simulink model "general_SD_model"  (R2021a)
settings: Solver=ode45  StartTime=0.0  StopTime=tfinal  FixedStep=T  MaxStep=0.01  RelTol=1e-12  AbsTol=1e-12  EnableMultiTasking=on
values from neighbouring files (symbols this model uses):
  position_amplitude = 0.03    [lab3_part_c.m]    (also in paramGen.m = 0.1; paramGenPartE.m = 0.15; part_c.m)
  position_offset = 0.15    [lab3_part_c.m]    (also in paramGen.m; paramGenPartE.m = 0.1; part_c.m)
  T = 0.001    [lab3_part_c.m]    (also in paramGen.m; paramGenPartE.m; part_c.m)
libraries: cstblocks x5
settings Model: OrderedModelArguments=off  Creator=cnielsen  LastModifiedBy=Daniel Robson
settings SolverCC: AutoScaleAbsTol=off  AlgebraicLoopSolver=TrustRegion
settings DataIOCC: SaveFormat=Array  SignalLoggingSaveFormat=ModelDataLogs  SaveOutput=off  SaveTime=off  ReturnWorkspaceOutputs=off  Refine=5
settings OptimizationCC: ExpressionDepthLimit=2147483647  LifeSpan=inf
settings DebuggingCC: UnderspecifiedInitializationDetection=Classic  MergeDetectMultiDrivingBlocksExec=none  SolverPrmCheckMsg=warning  FcnCallInpInsideContextMsg=warning  StateNameClashWarn=warning  SFUnexpectedBacktrackingDiag=warning  SFNoUnconditionalDefaultTransitionDiag=warning  SFExecutionAtInitializationDiag=none  SFMachineParentedDataDiag=warning  ArithmeticOperatorsInVariantConditions=warning
settings HardwareCC: ProdBitPerPointer=32  ProdBitPerSizeT=32  ProdBitPerPtrDiffT=32  ProdLargestAtomicFloat=None  ProdIntDivRoundTo=Undefined  ProdEndianess=Unspecified  ProdWordSize=32  ProdHWDeviceType=32-bit Generic
settings ModelReferenceCC: PropagateSignalLabelsOutOfModel=off
settings SFSimCC: SimUseLocalCustomCode=off  CustomCodeUndefinedFunction=UseInterfaceOnly
settings RTWCC: RTWUseLocalCustomCode=off
settings CodeAppCC: StateflowObjectComments=on
settings GRTTargetCC: TargetLangStandard=C89/C90 (ANSI)  CombineOutputUpdateFcns=off  GRTInterface=on
settings ConfigComp: CovMetricSettings=dw  CovSaveCumulativeToWorkspaceVar=on  CovSaveSingleToWorkspaceVar=on  CovExternalEMLEnable=off

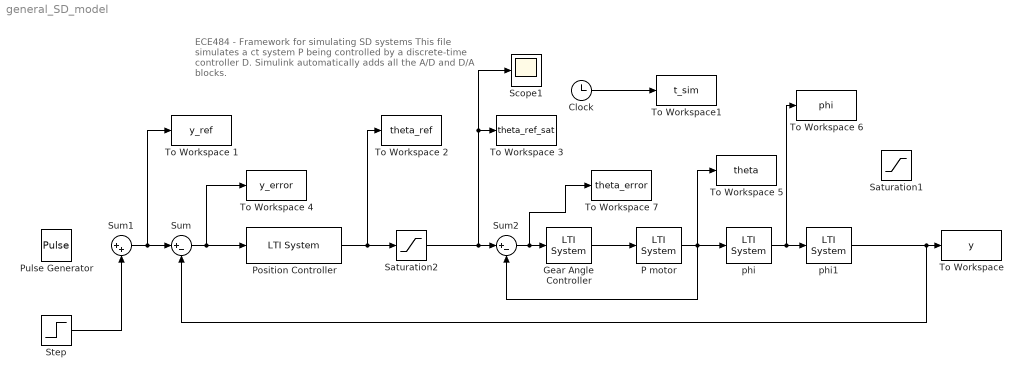
== system general_SD_model ==
  note: ECE484 - Framework for simulating SD systems
      | This file simulates a ct system P being controlled by a
      | discrete-time controller D. Simulink automatically adds all the
      | A/D and D/A blocks.
  Clock : Clock
  Gear Angle Controller : cstblocks/LTI System  sys=C_1  IC=[]
  P motor : cstblocks/LTI System  sys=P_motor  IC=[]
  Position Controller : cstblocks/LTI System  sys=C_2  IC=[]
  Pulse Generator : DiscretePulseGenerator  PulseType=Time based  Amplitude=position_amplitude  Period=20  PulseWidth=50  SampleTime=T
  Saturation1 : Saturate  UpperLimit=0.3916  LowerLimit=0
  Saturation2 : Saturate  UpperLimit=0.7  LowerLimit=-0.7
  Scope1 : Scope
  Step : Step  Time=0  After=position_offset  SampleTime=T
  Sum : Sum  Inputs=|+-
  Sum1 : Sum  Inputs=|++
  Sum2 : Sum  Inputs=|+-
  To Workspace : ToWorkspace  VariableName=y  SampleTime=T
  To Workspace 1 : ToWorkspace  VariableName=y_ref  SampleTime=T
  To Workspace 2 : ToWorkspace  VariableName=theta_ref  SampleTime=T
  To Workspace 3 : ToWorkspace  VariableName=theta_ref_sat  SampleTime=T
  To Workspace 4 : ToWorkspace  VariableName=y_error  SampleTime=T
  To Workspace 5 : ToWorkspace  VariableName=theta  SampleTime=T
  To Workspace 6 : ToWorkspace  VariableName=phi  SampleTime=T
  To Workspace 7 : ToWorkspace  VariableName=theta_error  SampleTime=T
  To Workspace1 : ToWorkspace  VariableName=t_sim  SampleTime=T
  phi : cstblocks/LTI System  sys=THETA_TO_PHI  IC=[]
  phi1 : cstblocks/LTI System  sys=PHI_TO_Y  IC=[]
  wires:
  Clock/1 -> To Workspace1/1
  Position Controller/1 -> To Workspace 2/1, Saturation2/1
  Gear Angle Controller/1 -> P motor/1
  Step/1 -> Sum1/2
  Sum1/1 -> To Workspace 1/1, Sum/1
  Sum/1 -> Position Controller/1, To Workspace 4/1
  Saturation2/1 -> Sum2/1, Scope1/1, To Workspace 3/1
  Sum2/1 -> To Workspace 7/1, Gear Angle Controller/1
  P motor/1 -> To Workspace 5/1, phi/1, Sum2/2
  phi/1 -> To Workspace 6/1, phi1/1
  phi1/1 -> Sum/2, To Workspace/1
